simulink model "AC_DC_POWER_SUPPLY"  (R2023a)
settings: Solver=VariableStepAuto  StartTime=0.0  StopTime=.4  RelTol=1e-3
libraries: spsThyristorLib x4, simulink x2, spsSeriesRLCBranchLib x2, spsVoltageMeasurementLib x2, spspowerguiLib x2, dspswit3 x1, spsACVoltageSourceLib x1
settings Model: Creator=Administrator  LastModifiedBy=user
settings SolverCC: AlgebraicLoopSolver=TrustRegion
settings DebuggingCC: UnconnectedInputMsg=warning  UnconnectedOutputMsg=warning  UnconnectedLineMsg=warning
settings ModelReferenceCC: EnableRefExpFcnMdlSchedulingChecks=on

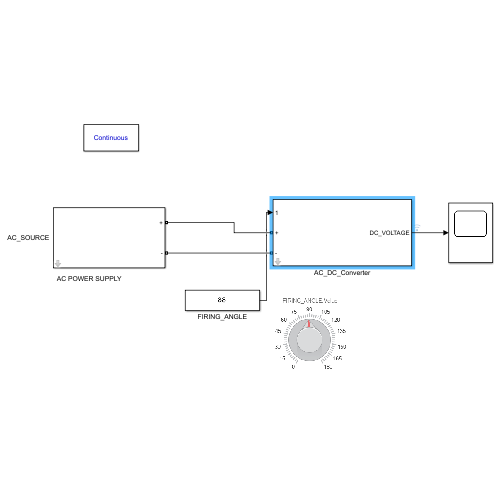
[thumbnail: Simulink's stored preview of the top-level diagram]
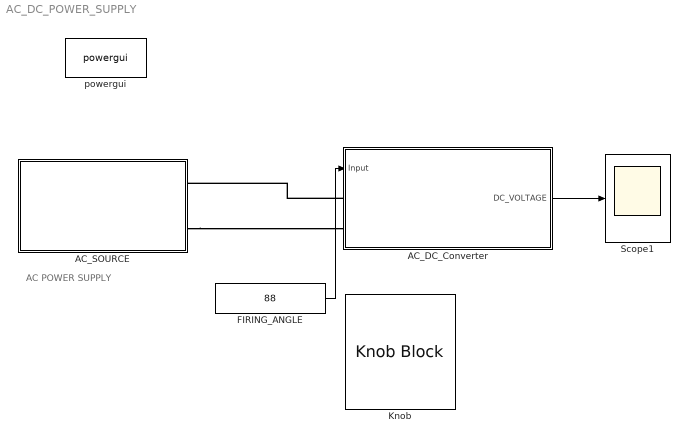
== system AC_DC_POWER_SUPPLY ==
  note: AC POWER SUPPLY
  AC_DC_Converter : Subsystem
      mask DialogControl DescGroupVar Prompt: AC/DC POWER SUPPLY
      mask DialogControl DescTextVar Prompt: transform the alternating current (AC) into a stable direct current (DC) voltage, which can then be used to power different electrical devices.
  AC_SOURCE : Subsystem  mask{AC=220, PHI=0}
      mask prompts: AC "Peak amplitude (V):"; PHI "Phase (deg):"
      mask DialogControl DescGroupVar Prompt: AC SOURCE
  FIRING_ANGLE : Constant  Value=88
  Knob : KnobBlock  ScaleMax=180
  Scope1 : Scope
  powergui : spspowerguiLib/powergui  Priority=1  SimulationMode=Continuous  SampleTime=50e-6  frequency=60  Iterations=50  frequencyindice=0  Pbase=100e6  ErrMax=1e-4  UnitsV=kV  UnitsW=MW  buscounter=0  FunctionMessages=off  echomessages=off  EnableUseOfTLC=off  CurrentSourceSwitches=off  DisableSnubberDevices=off  DisableRonSwitches=off  DisableVfSwitches=off  DisplayEquations=off  AutomaticDiscreteSolvers=off  SolverType=Tustin/Backward Euler (TBE)  Interpol=off  ExternalGateDelay=off  methode=off  Ts=100  x0status=blocks  SPID=on  SwTol=0  HookPort=off  NonlinearTolerance=1e-4  nMaxIteration=100  ContinueOnMaxIteration=off  RestoreLinks=warning  ResistiveCurrentMeasurement=off  Frange=[0:2:500]  Ylog=off  Xlog=on  ShowGrid=off  save=off  variable=ZData  structure=0  ZoomFFT=off  StartTime=0.0  cycles=1  DisplayStyle=1  fundamental=60  FreqAxis=off  MaxFrequency=1000  frequencyindicesteady=1  RmsSteady=1  display=off
  wires:
  FIRING_ANGLE/1 -> AC_DC_Converter/1(Input)
  AC_DC_Converter/1(DC_VOLTAGE) -> Scope1/1
  connections:
  AC_DC_Converter/LConn1 -- AC_SOURCE/RConn1
  AC_SOURCE/RConn2 -- AC_DC_Converter/LConn2

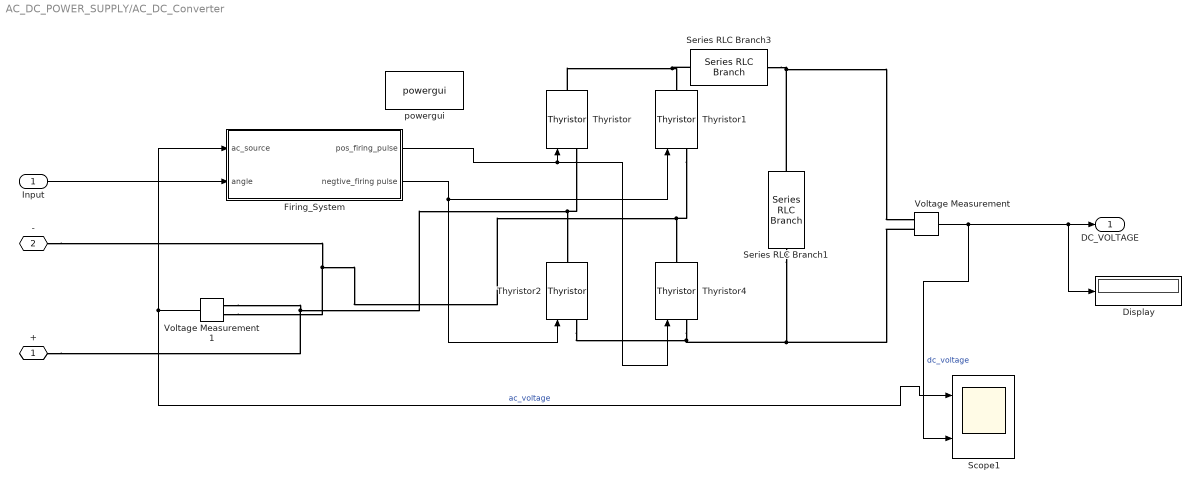
== system AC_DC_POWER_SUPPLY/AC_DC_Converter ==
  Input : Inport
  Display : Display
  Firing_System : Subsystem
  Scope1 : Scope  NumInputPorts=2
  Series RLC Branch1 : spsSeriesRLCBranchLib/Series RLC Branch  LConnTagsString=__new0  RConnTagsString=__new0  BranchType=C  Resistance=5  Inductance=1e-3  SetiL0=off  InitialCurrent=0  Capacitance=10e-6  Setx0=off  InitialVoltage=0  Measurements=None
  Series RLC Branch3 : spsSeriesRLCBranchLib/Series RLC Branch  LConnTagsString=__new0  RConnTagsString=__new0  BranchType=R  Resistance=40  Inductance=1e-3  SetiL0=off  InitialCurrent=0  Capacitance=10e-5  Setx0=off  InitialVoltage=0  Measurements=None
  Thyristor{,1..2,4} (4 alike) : spsThyristorLib/Thyristor  Ron=0.001  Lon=0  Vf=0.8  IC=0  Rs=500  Cs=250e-9  Measurements=off
  Voltage Measurement : spsVoltageMeasurementLib/Voltage Measurement  PhasorSimulation=off  OutputType=Complex  PSBequivalent=0
  Voltage Measurement1 : spsVoltageMeasurementLib/Voltage Measurement  PhasorSimulation=off  OutputType=Complex  PSBequivalent=0
  powergui : spspowerguiLib/powergui  Priority=1  SimulationMode=Continuous  SampleTime=50e-6  frequency=60  Iterations=50  frequencyindice=50  Pbase=100e6  ErrMax=1e-4  UnitsV=kV  UnitsW=MW  buscounter=0  FunctionMessages=off  echomessages=off  EnableUseOfTLC=off  CurrentSourceSwitches=off  DisableSnubberDevices=off  DisableRonSwitches=off  DisableVfSwitches=off  DisplayEquations=off  AutomaticDiscreteSolvers=off  SolverType=Tustin/Backward Euler (TBE)  Interpol=off  ExternalGateDelay=off  methode=off  Ts=100  x0status=blocks  SPID=on  SwTol=0  HookPort=off  NonlinearTolerance=1e-4  nMaxIteration=100  ContinueOnMaxIteration=off  RestoreLinks=warning  ResistiveCurrentMeasurement=off  Frange=[0:2:500]  Ylog=off  Xlog=on  ShowGrid=off  save=off  variable=ZData  structure=0  ZoomFFT=off  StartTime=0.0  cycles=1  DisplayStyle=1  fundamental=60  FreqAxis=off  MaxFrequency=1000  frequencyindicesteady=1  RmsSteady=1  display=off
  + : PMIOPort  Side=Left
  - : PMIOPort  Port=2  Side=Left
  DC_VOLTAGE : Outport
  wires:
  Voltage Measurement/1 -> Scope1/2, Display/1, DC_VOLTAGE/1  "dc_voltage"
  Firing_System/2(negtive_firing pulse) -> Thyristor1/1, Thyristor2/1
  Firing_System/1(pos_firing_pulse) -> Thyristor4/1, Thyristor/1
  Input/1 -> Firing_System/2(angle)
  Voltage Measurement1/1 -> Firing_System/1(ac_source), Scope1/1  "ac_voltage"
  connections:
  Thyristor1/LConn1 -- Voltage Measurement1/LConn2 -- -/RConn1 -- Thyristor4/RConn1
  Thyristor4/LConn1 -- Series RLC Branch1/RConn1 -- Voltage Measurement/LConn2 -- Thyristor2/LConn1
  Thyristor/LConn1 -- Voltage Measurement1/LConn1 -- +/RConn1 -- Thyristor2/RConn1
  Series RLC Branch1/LConn1 -- Series RLC Branch3/LConn1 -- Voltage Measurement/LConn1
  Thyristor/RConn1 -- Series RLC Branch3/RConn1 -- Thyristor1/RConn1

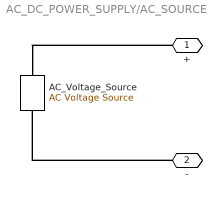
== system AC_DC_POWER_SUPPLY/AC_SOURCE ==
  AC_Voltage_Source : spsACVoltageSourceLib/AC Voltage Source  Amplitude=AC  Phase=PHI  Frequency=50  SampleTime=0  Measurements=None  BusType=swing  Pref=10e3  Qref=0  Qmin=-inf  Qmax=+inf
  + : PMIOPort  Side=Right
  - : PMIOPort  Port=2  Side=Right
  connections:
  +/RConn1 -- AC_Voltage_Source/RConn1
  -/RConn1 -- AC_Voltage_Source/LConn1

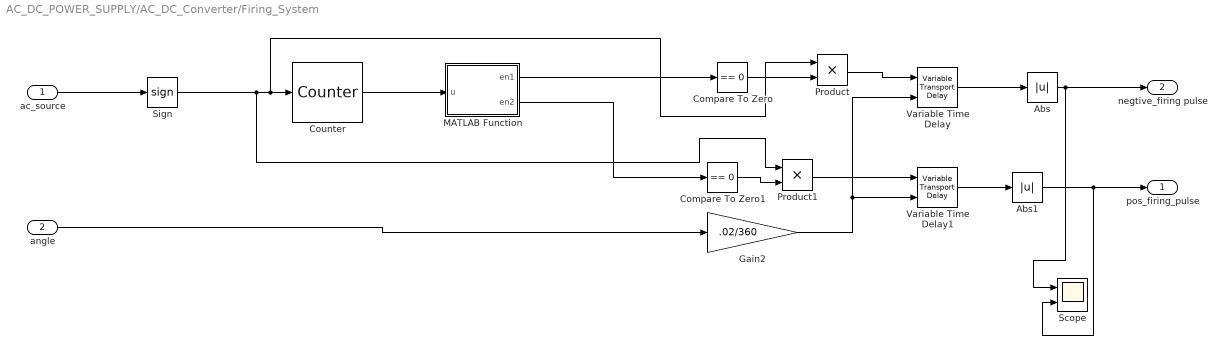
== system AC_DC_POWER_SUPPLY/AC_DC_Converter/Firing_System ==
  ac_source : Inport
  angle : Inport  Port=2
  Abs : Abs  SaturateOnIntegerOverflow=off
  Abs1 : Abs  SaturateOnIntegerOverflow=off
  Compare To Zero : simulink/Logic and Bit Operations/Compare To Zero  relop===  OutDataTypeStr=boolean
  Compare To Zero1 : simulink/Logic and Bit Operations/Compare To Zero  relop===  OutDataTypeStr=boolean
  Counter : dspswit3/Counter  Direction=Up  CountEvent=Either edge  CounterSize=User defined  MaxCount=255  InitialCount=0  Output=Count  HitValue=32  ResetInput=off  SamplesPerFrame=1  Ts=1  CntDtype=double  HitDtype=Logical
  Gain2 : Gain  Gain=.02/360
  MATLAB Function : MATLAB Function  TreatAsAtomicUnit=on
  Product : Product
  Product1 : Product
  Scope : Scope  NumInputPorts=2
  Sign : Signum
  Variable Time Delay : VariableTransportDelay  MaximumDelay=10
  Variable Time Delay1 : VariableTransportDelay  MaximumDelay=10
  pos_firing_pulse : Outport
  negtive_firing pulse : Outport  Port=2
  wires:
  Counter/1 -> MATLAB Function/1(u)
  MATLAB Function/1(en1) -> Compare To Zero/1
  Gain2/1 -> Variable Time Delay/2, Variable Time Delay1/2
  Variable Time Delay/1 -> Abs/1
  angle/1 -> Gain2/1
  MATLAB Function/2(en2) -> Compare To Zero1/1
  Sign/1 -> Product1/1, Product/1, Counter/1
  Variable Time Delay1/1 -> Abs1/1
  Abs/1 -> Scope/1, negtive_firing pulse/1
  Abs1/1 -> Scope/2, pos_firing_pulse/1
  ac_source/1 -> Sign/1
  Compare To Zero/1 -> Product/2
  Product/1 -> Variable Time Delay/1
  Compare To Zero1/1 -> Product1/2
  Product1/1 -> Variable Time Delay1/1

== matlab function AC_DC_POWER_SUPPLY/AC_DC_Converter/Firing_System/MATLAB Function ==
  data: u input; en1 output; en2 output
function [en1, en2] = fcn(u)
if rem(u, 2)==0
    en2 = 1;
    en1 = 0;
else
    en1 = 1;
    en2 = 0;
end
y = u;
